simulink model "soc_dvbs2_top"  (R2025b)
settings: Solver=VariableStepAuto  StartTime=0.0  StopTime=0.3  RelTol=1e-3
PreLoadFcn:
  | RxFrameSize = 2048;
  | soc_dvbs2_init;
InitFcn:
  | RxFrameSize = 2048;
  | soc_dvbs2_init;
model workspace (MAT data in the model file):
  mmap = soc.memmap.MemoryMap
  mmap.isMapValid = 1
  mmap.controllerInfo = soc.memmap.MemController
  mmap.controllerInfo.memPSRange = {'2', 'G'}
  mmap.controllerInfo.memPLBaseAddr = '0x500000000'
  mmap.controllerInfo.memPLRange = {'4', 'G'}
  mmap.controllerInfo.memPLBaseAddrMMU = {9, '0'}
  mmap.controllerInfo.regBaseAddr = '0xA0000000'
  mmap.controllerInfo.regAddrRange = {'256', 'M'}
  mmap.map(1) = soc.memmap.MapParams
  mmap.map(1).type = 'PS Memory Region'
  mmap.map(1).name = 'AXI4-Stream to Software'
  mmap.map(1).baseAddr = '0x00000000'
  mmap.map(1).range = {'32', 'K'}
  mmap.map(1).path = 'soc_dvbs2_top/AXI4-Stream to Software'
  mmap.map(2) = soc.memmap.MapParams
  mmap.map(2).type = 'User Component'
  mmap.map(2).name = 'DVBS2'
  mmap.map(2).baseAddr = '0xA0000000'
  mmap.map(2).range = {'64', 'K'}
  mmap.map(2).path = 'soc_dvbs2_fpga/DVBS2'
  mmap.map(2).regs(1) = soc.memmap.IPCoreRegParams
  mmap.map(2).regs(1).register = 'HDL Coder registers'
  mmap.map(2).regs(1).offset = '0x0000 - 0x00FF'
  mmap.map(2).regs(1).vectorlength = 'N/A'
  mmap.map(2).regs(1).type = 'Reserved'
  mmap.map(2).regs(1).reserved = 1
  mmap.map(2).regs(2) = soc.memmap.IPCoreRegParams
  mmap.map(2).regs(2).blkname = 'DVBS2'
  mmap.map(2).regs(2).register = 'nframesSynced'
  mmap.map(2).regs(2).offset = '0x0100'
  mmap.map(2).regs(2).vectorlength = '1'
  mmap.map(2).regs(2).type = 'Processor read channel'
  mmap.map(2).regs(3) = soc.memmap.IPCoreRegParams
  mmap.map(2).regs(3).blkname = 'DVBS2'
  mmap.map(2).regs(3).register = 'decodedModcod'
  mmap.map(2).regs(3).offset = '0x0104'
  mmap.map(2).regs(3).vectorlength = '1'
  mmap.map(2).regs(3).type = 'Processor read channel'
  mmap.map(2).regs(4) = soc.memmap.IPCoreRegParams
  mmap.map(2).regs(4).blkname = 'DVBS2'
  mmap.map(2).regs(4).register = 'decodedFecFrame'
  mmap.map(2).regs(4).offset = '0x0108'
  mmap.map(2).regs(4).vectorlength = '1'
  mmap.map(2).regs(4).type = 'Processor read channel'
  mmap.map(2).regs(5) = soc.memmap.IPCoreRegParams
  mmap.map(2).regs(5).blkname = 'DVBS2'
  mmap.map(2).regs(5).register = 'FreqEst'
  mmap.map(2).regs(5).offset = '0x010C'
  mmap.map(2).regs(5).vectorlength = '1'
  mmap.map(2).regs(5).type = 'Processor read channel'
  mmap.map(2).regs(6) = soc.memmap.IPCoreRegParams
  mmap.map(2).regs(6).blkname = 'DVBS2'
  mmap.map(2).regs(6).register = 'TSorGS'
  mmap.map(2).regs(6).offset = '0x0110'
  mmap.map(2).regs(6).vectorlength = '1'
  mmap.map(2).regs(6).type = 'Processor read channel'
  mmap.map(2).regs(7) = soc.memmap.IPCoreRegParams
  mmap.map(2).regs(7).blkname = 'DVBS2'
  mmap.map(2).regs(7).register = 'UPL'
  mmap.map(2).regs(7).offset = '0x0114'
  mmap.map(2).regs(7).vectorlength = '1'
  mmap.map(2).regs(7).type = 'Processor read channel'
  mmap.map(2).regs(8) = soc.memmap.IPCoreRegParams
  mmap.map(2).regs(8).blkname = 'DVBS2'
  mmap.map(2).regs(8).register = 'DFL'
  mmap.map(2).regs(8).offset = '0x0118'
  mmap.map(2).regs(8).vectorlength = '1'
  mmap.map(2).regs(8).type = 'Processor read channel'
  mmap.map(2).regs(9) = soc.memmap.IPCoreRegParams
  mmap.map(2).regs(9).blkname = 'DVBS2'
  mmap.map(2).regs(9).register = 'SYNC'
  mmap.map(2).regs(9).offset = '0x011C'
  mmap.map(2).regs(9).vectorlength = '1'
  mmap.map(2).regs(9).type = 'Processor read channel'
  mmap.map(2).regs(10) = soc.memmap.IPCoreRegParams
  mmap.map(2).regs(10).blkname = 'DVBS2'
  mmap.map(2).regs(10).register = 'nbitsErrored'
  mmap.map(2).regs(10).offset = '0x0120'
  mmap.map(2).regs(10).vectorlength = '1'
  mmap.map(2).regs(10).type = 'Processor read channel'
  mmap.map(2).regs(11) = soc.memmap.IPCoreRegParams
  mmap.map(2).regs(11).blkname = 'DVBS2'
  mmap.map(2).regs(11).register = 'nbitsReceived'
  mmap.map(2).regs(11).offset = '0x0124'
  mmap.map(2).regs(11).vectorlength = '1'
  mmap.map(2).regs(11).type = 'Processor read channel'
  mmap.map(2).regs(12) = soc.memmap.IPCoreRegParams
  mmap.map(2).regs(12).blkname = 'DVBS2'
  mmap.map(2).regs(12).register = 'adc_dac_loopback'
  mmap.map(2).regs(12).offset = '0x0128'
  mmap.map(2).regs(12).vectorlength = '1'
  mmap.map(2).regs(12).type = 'Processor write channel'
  mmap.map(2).regs(13) = soc.memmap.IPCoreRegParams
  mmap.map(2).regs(13).blkname = 'DVBS2'
  mmap.map(2).regs(13).register = 'enbNoise'
  mmap.map(2).regs(13).offset = '0x012C'
  mmap.map(2).regs(13).vectorlength = '1'
  mmap.map(2).regs(13).type = 'Processor write channel'
  mmap.map(2).regs(14) = soc.memmap.IPCoreRegParams
  mmap.map(2).regs(14).blkname = 'DVBS2'
  mmap.map(2).regs(14).register = 'snrdB'
  mmap.map(2).regs(14).offset = '0x0130'
  mmap.map(2).regs(14).vectorlength = '1'
  mmap.map(2).regs(14).type = 'Processor write channel'
  mmap.map(2).regs(15) = soc.memmap.IPCoreRegParams
  mmap.map(2).regs(15).blkname = 'DVBS2'
  mmap.map(2).regs(15).register = 'CFO'
  mmap.map(2).regs(15).offset = '0x0134'
  mmap.map(2).regs(15).vectorlength = '1'
  mmap.map(2).regs(15).type = 'Processor write channel'
  mmap.map(2).regs(16) = soc.memmap.IPCoreRegParams
  mmap.map(2).regs(16).blkname = 'DVBS2'
  mmap.map(2).regs(16).register = 'CPO'
  mmap.map(2).regs(16).offset = '0x0138'
  mmap.map(2).regs(16).vectorlength = '1'
  mmap.map(2).regs(16).type = 'Processor write channel'
  mmap.map(2).regs(17) = soc.memmap.IPCoreRegParams
  mmap.map(2).regs(17).blkname = 'DVBS2'
  mmap.map(2).regs(17).register = 'modcodIdx'
  mmap.map(2).regs(17).offset = '0x013C'
  mmap.map(2).regs(17).vectorlength = '1'
  mmap.map(2).regs(17).type = 'Processor write channel'
  mmap.map(2).regs(18) = soc.memmap.IPCoreRegParams
  mmap.map(2).regs(18).blkname = 'DVBS2'
  mmap.map(2).regs(18).register = 'resetFCPO'
  mmap.map(2).regs(18).offset = '0x0140'
  mmap.map(2).regs(18).vectorlength = '1'
  mmap.map(2).regs(18).type = 'Processor write channel'
  mmap.map(2).regs(19) = soc.memmap.IPCoreRegParams
  mmap.map(2).regs(19).blkname = 'DVBS2'
  mmap.map(2).regs(19).register = 'resetDisplay'
  mmap.map(2).regs(19).offset = '0x0144'
  mmap.map(2).regs(19).vectorlength = '1'
  mmap.map(2).regs(19).type = 'Processor write channel'
  mmap.map(3) = soc.memmap.MapParams
  mmap.map(3).type = 'Implicit Component'
  mmap.map(3).name = 'AXI4-Stream to Software DMA S2MM'
  mmap.map(3).baseAddr = '0xA0010000'
  mmap.map(3).range = {'64', 'K'}
  mmap.map(4) = soc.memmap.MapParams
  mmap.map(4).type = 'Implicit Component'
  mmap.map(4).name = 'RFDataConverter/s_axi'
  mmap.map(4).baseAddr = '0xA3C00000'
  mmap.map(4).range = {'256', 'K'}
  mwTaskManagerKernelLatency = 0
  socicb{1}.Registry = containers.Map
  socicb{1}.Registry.serialization.keys = {45989.0006104}
  socicb{1}.Registry.serialization.values = {1}
  socicb{1}.Registry.serialization.uniformity = 0
  socicb{1}.Registry.serialization.keyType = 'double'
  socicb{1}.Registry.serialization.valueType = 'any'
  socicb{1}.Index = 2
  socicb{2}.Registry = containers.Map
  socicb{2}.Registry.serialization.keys = {}
  socicb{2}.Registry.serialization.values = {}
  socicb{2}.Registry.serialization.uniformity = 0
  socicb{2}.Registry.serialization.keyType = 'double'
  socicb{2}.Registry.serialization.valueType = 'any'
  socicb{2}.Index = 1
  socvcb = containers.Map
  socvcb.serialization.keys = {2.00012207031, 2.00024414062, 2.00036621094, 3.00012207031, 3.00036621094, 3.00061035156, 3.00073242188, 3.00109863281, 3.00158691406, 3.00219726562, 3.00329589844, 3.00366210938, 3.00939941406, 3.01062011719, 3.02478027344, 3.02746582031, 3.0302734375, 3.03332519531, 3.09558105469, 4.00012207031, 4.00024414062, 4.00036621094, 4.00061035156, 4.00073242188, 4.00109863281, 4.00122070312, 4.00183105469, 4.00891113281, 4.00915527344, 4.0244140625, 4.02673339844, 4.02807617188, 4.03259277344, 4.36804199219, 5.00061035156, 5.00073242188, 5.00122070312, 5.00134277344, 5.00891113281, 5.00915527344, 5.02429199219, 5.02648925781, 5.02734375, 5.03234863281, 154.00012207, 154.044311523, 154.045654297, 154.083618164, 154.113647461, 154.172729492, 155.003417969, 356.163696289, 514.000244141, 515.381347656, 515.829833984, 1542.00634766, 2562.56542969, 15856.0009766, 15857.0006104, 15858.0004883, 17279.0084229, 17280.0084229, 44819.0001221, 45026.0063477, 45722.0001221}
  socvcb.serialization.values : function handle (value not decoded)
  socvcb.serialization.uniformity = 0
  socvcb.serialization.keyType = 'double'
  socvcb.serialization.valueType = 'any'
values from neighbouring files (symbols this model uses):
  fs = Rsym *32    (= 128000000)    [soc_dvbs2_init.m]
undefined symbols (not defined in the file or in its folder): D1, Fs, I, m, n, P, Q
libraries: socmemlib x2, prociodatalib x2, hostiolib x2, proctasklib x1, xilinxrfsoclib x1
CloseFcn:
  | h = warning('off','MATLAB:rmpath:DirNotFound');
  | rmpath(fullfile(matlabroot,'toolbox','whdl','whdlexamples','whdlexamples'));
  | warning(h);
  | clear h;
settings Model: DataDictionary=dvbs2hdlReceiverData.sldd  SimulationMode=accelerator  Creator=The MathWorks, Inc.  LastModifiedBy=The MathWorks, Inc.
settings SolverCC: AlgebraicLoopSolver=TrustRegion  PositivePriorityOrder=on  AutoInsertRateTranBlk=on  MaxZcPerStep=1.0
settings DataIOCC: SaveFormat=StructureWithTime  ReturnWorkspaceOutputs=off
settings OptimizationCC: BlockReduction=off  ConditionallyExecuteInputs=off  DefaultParameterBehavior=Inlined  ReuseModelBlockBuffer=off  PassReuseOutputArgsAs=Individual arguments  MaxStackSize=64  EfficientTunableParamExpr=on
settings DebuggingCC: AlgebraicLoopMsg=error  SingleTaskRateTransMsg=error  IntegerOverflowMsg=none  ParameterPrecisionLossMsg=none  ParameterTunabilityLossMsg=error  UnconnectedInputMsg=warning  UnconnectedOutputMsg=warning  UnconnectedLineMsg=warning  SubsystemReferenceDiagnosticForUnitTest=warning  ArithmeticOperatorsInVariantConditions=warning
settings HardwareCC: ProdBitPerLong=64.0  ProdLargestAtomicInteger=LongLong  ProdLargestAtomicFloat=Double  ProdLongLongMode=on  ProdHWDeviceType=ARM Compatible->ARM Cortex-A (64-bit)  HardwareBoardFeatureSet=SoCBlockset
settings ModelReferenceCC: EnableRefExpFcnMdlSchedulingChecks=on  ModelReferenceNumInstancesAllowed=Single
settings SFSimCC: SimUseLocalCustomCode=off  CustomCodeUndefinedFunction=UseInterfaceOnly
settings RTWCC: SystemTargetFile=ert.tlc  HardwareBoard=Xilinx Zynq UltraScale+ RFSoC ZCU111 Evaluation Kit  TLCOptions="-aInlineSetEventsForThisBaseRateFcn=TLC_FALSE -aSuppressMultiTaskScheduler=TLC_FALSE  -aRateBasedStepFcn=0"  TemplateMakefile=ert_default_tmf  GenerateReport=on  RTWUseLocalCustomCode=off  Toolchain=Linaro AArch64 Linux v6.3.1  IncludeHyperlinkInReport=on  LaunchReport=on  GenerateTraceInfo=on  GenerateTraceReport=on  GenerateTraceReportSl=on  GenerateTraceReportSf=on  GenerateTraceReportEml=on  GPUComputeCapability=3.5  DLArmComputeVersion=19.05  Description=Embedded Coder
settings CodeAppCC: ForceParamTrailComments=on  IgnoreCustomStorageClasses=off  OperatorAnnotations=on  SimulinkDataObjDesc=on  SFDataObjDesc=on  InsertBlockDesc=on
settings ERTTargetCC: InlinedParameterPlacement=Hierarchical

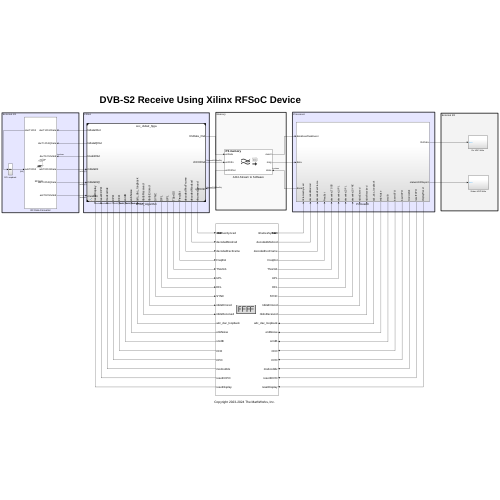
[thumbnail: Simulink's stored preview of the top-level diagram]
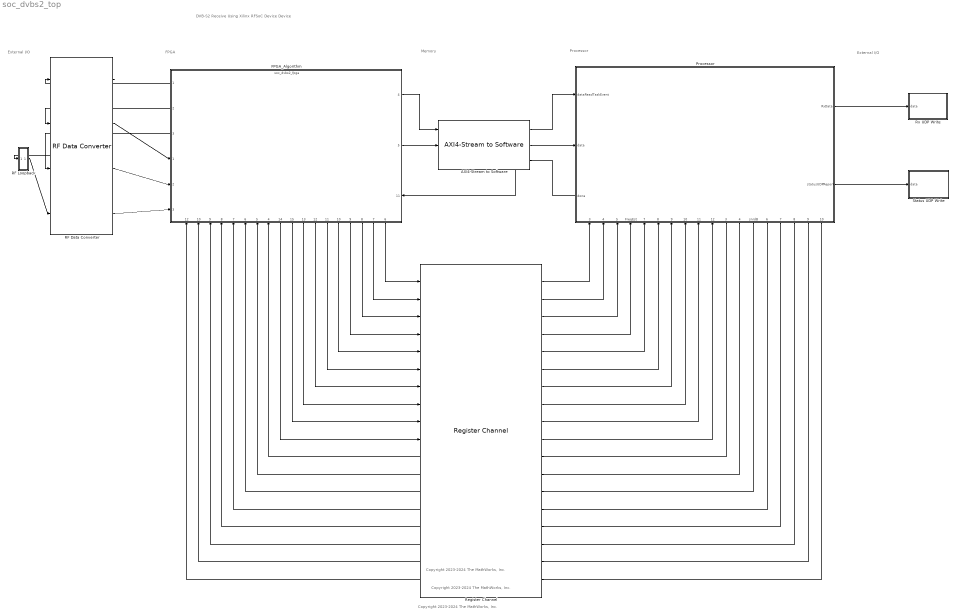
== system soc_dvbs2_top ==
  note: FPGA
  note: Memory
  note: Processor
  note: Copyright 2023-2024 The MathWorks, Inc.
  note: External I/O
  note: External I/O
  note: DVB-S2 Receive Using Xilinx RFSoC Device Device
  note: Copyright 2023-2024 The MathWorks, Inc.
  note: Copyright 2023-2024 The MathWorks, Inc.
  AXI4-Stream to Software : socmemlib/AXI4-Stream to Software  MemorySimulation=Burst accurate  MemorySelection=PS memory  MRNumBuffers=4  BurstLengthWriterChIf=256  FIFODepthWriter=8  FIFOAFullDepthWriter=6  ICClockFrequencyWriter=100  ICDataWidthWriter=64  ChDimensionsWriterChIf=1  ChTypeWriterChIf=uint32  ChFrameSampleTimeWriterChIf=1/fs  ChBitPackedWriterChIf=off  ChDimensionsReaderChIf=RxFrameSize  ChTypeReaderChIf=uint32  LastTargetBoard=Xilinx Zynq UltraScale+ RFSoC ZCU111 Evaluation Kit  MRRegionSize=32768  MRBufferSize=8192  DiagnosticLevel=No debug
  FPGA_Algorithm : ModelReference  ModelNameDialog=soc_dvbs2_fpga.slx  ModelReferenceVersion=9.0
      settings: PortSchema="{\"entries\":[{\"content\":{\"sides\":[{\"content\":{\"connectorIds\":[\"Out1\",\"Out2\",\"Out3\",\"In1\",\"In2\",\"In3\"]},\"type\":\"ConnectorPlacement.EquallySpacedRectSide\",\"uuid\":\"5a98e095-40d9-43f8-91e5-a805a03516fd\"},{\"content\":{\"connectorIds\":[\"Out4\",\"Out5\",\"In11\"],\"side\":\"RIGHT\"},\"type\":\"ConnectorPlacement.EquallySpacedRectSide\",\"uuid\":\"242f1ec7-c947-482c-82ab-d4fa225331bb\"},{\"content\":{\"side\":\"TOP\"},\"type\":\"ConnectorPlacement.EquallySpacedRectSide\",\"uuid\":\"d3f55be4-91f3-4b02-af75-0bf7e7e1b925\"},{\"content\":{\"connectorIds\":[\"In12\",\"In10\",\"In9\",\"In8\",\"In7\",\"In6\",\"In5\",\"In4\",\"Out14\",\"Out15\",\"Out13\",\"Out12\",\"Out11\",\"Out10\",\"Out9\",\"Out8\",\"Out7\",\"Out6\"],\"side\":\"BOTTOM\"},\"type\":\"ConnectorPlacement.EquallySpacedRectSide\",\"uuid\":\"11ee90da-1deb-4c1f-bd41-f9aa9c63736b\"}]},\"type\":\"ConnectorPlacement.EquallySpacedConnector\",\"uuid\":\"1ac0077b-1539-4750-8893-00c30e797fc3\"}],\"packageUris\":[\"http://schema.mathworks.com/mf0/Connector/R2020b\"],\"version\":\"1.0\"}"
  Processor : Subsystem
      settings: PortSchema="{\"entries\":[{\"content\":{\"sides\":[{\"content\":{\"connectorIds\":[\"In1\",\"In2\",\"Out11\"]},\"type\":\"ConnectorPlacement.EquallySpacedRectSide\",\"uuid\":\"19674b72-8bc7-450a-aa32-317c951772fa\"},{\"content\":{\"connectorIds\":[\"Out1\",\"Out2\"],\"side\":\"RIGHT\"},\"type\":\"ConnectorPlacement.EquallySpacedRectSide\",\"uuid\":\"8c37c977-a2a8-45d5-9785-0385e2fd1bd5\"},{\"content\":{\"side\":\"TOP\"},\"type\":\"ConnectorPlacement.EquallySpacedRectSide\",\"uuid\":\"969f5835-0601-41e1-8044-5c28f455717a\"},{\"content\":{\"connectorIds\":[\"In3\",\"In4\",\"In5\",\"In6\",\"In7\",\"In8\",\"In9\",\"In10\",\"In11\",\"In12\",\"Out3\",\"Out4\",\"Out5\",\"Out6\",\"Out7\",\"Out8\",\"Out9\",\"Out10\"],\"side\":\"BOTTOM\"},\"type\":\"ConnectorPlacement.EquallySpacedRectSide\",\"uuid\":\"78263d19-cd7e-4a64-923d-d1623dce68f9\"}]},\"type\":\"ConnectorPlacement.EquallySpacedConnector\",\"uuid\":\"9dca4fc9-649f-4a7f-a81c-0545d597adf9\"}],\"packageUris\":[\"http://schema.mathworks.com/mf0/Connector/R2020b\"],\"version\":\"1.0\"}"
  RF Data Converter : xilinxrfsoclib/RF Data Converter  RFDCSim=Pass-through  tabPromptsCB=0  RFInterface=Customize  digitalInterface=I/Q  dac11Enable=off  dac12Enable=off  dac13Enable=off  dac14Enable=off  dac21Enable=off  dac22Enable=off  dac23Enable=on  dac24Enable=off  dac31Enable=off  dac32Enable=off  dac33Enable=off  dac34Enable=off  dac41Enable=off  dac42Enable=off  dac43Enable=off  dac44Enable=off  matchDACParam=on  dacSampleRate=2048  dacDatapathMode=Full Nyquist (0 to Fs/2)  interpolationMode=4  dacSamplesPerCycle=4  dacMixerType=Fine  dacMixerMode=I/Q->Real  dacMixerFrequency=Fs/2  dacNCOFrequency=[0.860]  dacNCOPhase=[0]  invertSyncFilter=off  dacTile1SampleRate=1000  dac11DatapathMode=Full Nyquist (0 to Fs/2)  dac11InterpolationMode=2  dac11SamplesPerCycle=2  dac11MixerType=Coarse  dac11MixerMode=I/Q->Real  dac11MixerFrequency=Fs/2  dac11NCOFrequency=0  dac11NCOPhase=0  dac11InvertSyncFilter=off  dac12DatapathMode=Full Nyquist (0 to Fs/2)  dac12InterpolationMode=2  dac12SamplesPerCycle=2  dac12MixerType=Coarse  dac12MixerMode=I/Q->Real  dac12MixerFrequency=Fs/2  dac12NCOFrequency=0  dac12NCOPhase=0  dac12InvertSyncFilter=off  dac13DatapathMode=Full Nyquist (0 to Fs/2)  dac13InterpolationMode=2  dac13SamplesPerCycle=2  dac13MixerType=Coarse  dac13MixerMode=I/Q->Real  dac13MixerFrequency=Fs/2  dac13NCOFrequency=0  dac13NCOPhase=0  dac13InvertSyncFilter=off  dac14DatapathMode=Full Nyquist (0 to Fs/2)  dac14InterpolationMode=2  dac14SamplesPerCycle=2  dac14MixerType=Coarse  dac14MixerMode=I/Q->Real  dac14MixerFrequency=Fs/2  dac14NCOFrequency=0  dac14NCOPhase=0  dac14InvertSyncFilter=off  dacTile2SampleRate=1000  dac21DatapathMode=Full Nyquist (0 to Fs/2)  dac21InterpolationMode=2  dac21SamplesPerCycle=2  dac21MixerType=Coarse  dac21MixerMode=I/Q->Real  dac21MixerFrequency=Fs/2  dac21NCOFrequency=0  dac21NCOPhase=0  dac21InvertSyncFilter=off  dac22DatapathMode=Full Nyquist (0 to Fs/2)  dac22InterpolationMode=2  dac22SamplesPerCycle=2  dac22MixerType=Coarse  dac22MixerMode=I/Q->Real  dac22MixerFrequency=Fs/2  dac22NCOFrequency=0  dac22NCOPhase=0  dac22InvertSyncFilter=off  dac23DatapathMode=Full Nyquist (0 to Fs/2)  dac23InterpolationMode=2  dac23SamplesPerCycle=2  dac23MixerType=Coarse  dac23MixerMode=I/Q->Real  dac23MixerFrequency=Fs/2  dac23NCOFrequency=0  dac23NCOPhase=0  dac23InvertSyncFilter=off  dac24DatapathMode=Full Nyquist (0 to Fs/2)  dac24InterpolationMode=2  dac24SamplesPerCycle=2  dac24MixerType=Coarse  dac24MixerMode=I/Q->Real  dac24MixerFrequency=Fs/2  dac24NCOFrequency=0  dac24NCOPhase=0  dac24InvertSyncFilter=off  dacTile3SampleRate=1000  dac31DatapathMode=Full Nyquist (0 to Fs/2)  dac31InterpolationMode=2  dac31SamplesPerCycle=2  dac31MixerType=Coarse  dac31MixerMode=I/Q->Real  dac31MixerFrequency=Fs/2  dac31NCOFrequency=0  dac31NCOPhase=0  dac31InvertSyncFilter=off  dac32DatapathMode=Full Nyquist (0 to Fs/2)  dac32InterpolationMode=2  dac32SamplesPerCycle=2  dac32MixerType=Coarse  dac32MixerMode=I/Q->Real  dac32MixerFrequency=Fs/2  dac32NCOFrequency=0  dac32NCOPhase=0  dac32InvertSyncFilter=off  dac33DatapathMode=Full Nyquist (0 to Fs/2)  dac33InterpolationMode=2  dac33SamplesPerCycle=2  dac33MixerType=Coarse  dac33MixerMode=I/Q->Real  dac33MixerFrequency=Fs/2  dac33NCOFrequency=0  dac33NCOPhase=0  dac33InvertSyncFilter=off  dac34DatapathMode=Full Nyquist (0 to Fs/2)  dac34InterpolationMode=2  dac34SamplesPerCycle=2  dac34MixerType=Coarse  dac34MixerMode=I/Q->Real  dac34MixerFrequency=Fs/2  dac34NCOFrequency=0  dac34NCOPhase=0  dac34InvertSyncFilter=off  dacTile4SampleRate=1000  dac41DatapathMode=Full Nyquist (0 to Fs/2)  dac41InterpolationMode=2  dac41SamplesPerCycle=2  dac41MixerType=Coarse  dac41MixerMode=I/Q->Real  dac41MixerFrequency=Fs/2  dac41NCOFrequency=0  dac41NCOPhase=0  dac41InvertSyncFilter=off  dac42DatapathMode=Full Nyquist (0 to Fs/2)  dac42InterpolationMode=2  dac42SamplesPerCycle=2  dac42MixerType=Coarse  dac42MixerMode=I/Q->Real  dac42MixerFrequency=Fs/2  dac42NCOFrequency=0  dac42NCOPhase=0  dac42InvertSyncFilter=off  dac43DatapathMode=Full Nyquist (0 to Fs/2)  dac43InterpolationMode=2  dac43SamplesPerCycle=2  dac43MixerType=Coarse  dac43MixerMode=I/Q->Real  dac43MixerFrequency=Fs/2  dac43NCOFrequency=0  dac43NCOPhase=0  dac43InvertSyncFilter=off  dac44DatapathMode=Full Nyquist (0 to Fs/2)  dac44InterpolationMode=2  dac44SamplesPerCycle=2  dac44MixerType=Coarse  dac44MixerMode=I/Q->Real  dac44MixerFrequency=Fs/2  dac44NCOFrequency=0  dac44NCOPhase=0  dac44InvertSyncFilter=off  adc11Enable=on  adc12Enable=off  adc13Enable=off  adc14Enable=off  adc21Enable=off  adc22Enable=off  adc23Enable=off  adc24Enable=off  adc31Enable=off  adc32Enable=off  adc33Enable=off  adc34Enable=off  adc41Enable=off  adc42Enable=off  adc43Enable=off  adc44Enable=off  adcOutUnpackedData=on  matchADCParam=on  adcSampleRate=2048  decimationMode=4  adcSamplesPerCycle=4  adcMixerType=Fine  adcMixerMode=Real->I/Q  adcMixerFrequency=Fs/2  adcNCOFrequency=[-0.860]  adcNCOPhase=[0]  adcTile1SampleRate=1000  adc11DecimationMode=2  adc11SamplesPerCycle=2  adc11MixerType=Coarse  adc11MixerMode=Real->I/Q  adc11MixerFrequency=Fs/2  adc11NCOFrequency=0  adc11NCOPhase=0  adc12DecimationMode=2  adc12SamplesPerCycle=2  adc12MixerType=Coarse  adc12MixerMode=Real->I/Q  adc12MixerFrequency=Fs/2  adc12NCOFrequency=0  adc12NCOPhase=0  adc13DecimationMode=2  adc13SamplesPerCycle=2  adc13MixerType=Coarse  adc13MixerMode=Real->I/Q  adc13MixerFrequency=Fs/2  adc13NCOFrequency=0  adc13NCOPhase=0  adc14DecimationMode=2  adc14SamplesPerCycle=2  adc14MixerType=Coarse  adc14MixerMode=Real->I/Q  adc14MixerFrequency=Fs/2  adc14NCOFrequency=0  adc14NCOPhase=0  adcTile2SampleRate=1000  adc21DecimationMode=2  adc21SamplesPerCycle=2  adc21MixerType=Coarse  adc21MixerMode=Real->I/Q  adc21MixerFrequency=Fs/2  adc21NCOFrequency=0  adc21NCOPhase=0  adc22DecimationMode=2  adc22SamplesPerCycle=2  adc22MixerType=Coarse  adc22MixerMode=Real->I/Q  adc22MixerFrequency=Fs/2  adc22NCOFrequency=0  adc22NCOPhase=0  adc23DecimationMode=2  adc23SamplesPerCycle=2  adc23MixerType=Coarse  adc23MixerMode=Real->I/Q  adc23MixerFrequency=Fs/2  adc23NCOFrequency=0  adc23NCOPhase=0  adc24DecimationMode=2  adc24SamplesPerCycle=2  adc24MixerType=Coarse  adc24MixerMode=Real->I/Q  adc24MixerFrequency=Fs/2  adc24NCOFrequency=0  adc24NCOPhase=0  adcTile3SampleRate=1000  adc31DecimationMode=2  adc31SamplesPerCycle=2  adc31MixerType=Coarse  adc31MixerMode=Real->I/Q  adc31MixerFrequency=Fs/2  adc31NCOFrequency=0  adc31NCOPhase=0  adc32DecimationMode=2  adc32SamplesPerCycle=2  adc32MixerType=Coarse  adc32MixerMode=Real->I/Q  adc32MixerFrequency=Fs/2  adc32NCOFrequency=0  adc32NCOPhase=0  adc33DecimationMode=2  adc33SamplesPerCycle=2  adc33MixerType=Coarse  adc33MixerMode=Real->I/Q  adc33MixerFrequency=Fs/2  adc33NCOFrequency=0  adc33NCOPhase=0  adc34DecimationMode=2  adc34SamplesPerCycle=2  adc34MixerType=Coarse  adc34MixerMode=Real->I/Q  adc34MixerFrequency=Fs/2  adc34NCOFrequency=0  adc34NCOPhase=0  adcTile4SampleRate=1000  adc41DecimationMode=2  adc41SamplesPerCycle=2  adc41MixerType=Coarse  adc41MixerMode=Real->I/Q  adc41MixerFrequency=Fs/2  adc41NCOFrequency=0  adc41NCOPhase=0  adc42DecimationMode=2  adc42SamplesPerCycle=2  adc42MixerType=Coarse  adc42MixerMode=Real->I/Q  adc42MixerFrequency=Fs/2  adc42NCOFrequency=0  adc42NCOPhase=0  adc43DecimationMode=2  adc43SamplesPerCycle=2  adc43MixerType=Coarse  adc43MixerMode=Real->I/Q  adc43MixerFrequency=Fs/2  adc43NCOFrequency=0  adc43NCOPhase=0  adc44DecimationMode=2  adc44SamplesPerCycle=2  adc44MixerType=Coarse  adc44MixerMode=Real->I/Q  adc44MixerFrequency=Fs/2  adc44NCOFrequency=0  adc44NCOPhase=0  multiTileSync=off  externalPLL=off  dacRealTimeNCOPortsEnable=off  adcRealTimeNCOPortsEnable=off  adcRealTimePortsEnable=off  adcThresholdMode=Sticky over  adcThreshold1=0  adcDelayCounter=0  adcThreshold2Mode=Sticky over  adcThreshold2=0  adcThreshold2DelayCounter=0  adc11ThresholdMode=Sticky over  adc11Threshold1=0  adc11DelayCounter=0  adc11Threshold2Mode=Sticky over  adc11Threshold2=0  adc11Threshold2DelayCounter=0  adc12ThresholdMode=Sticky over  adc12Threshold1=0  adc12DelayCounter=0  adc12Threshold2Mode=Sticky over  adc12Threshold2=0  adc12Threshold2DelayCounter=0  adc13ThresholdMode=Sticky over  adc13Threshold1=0  adc13DelayCounter=0  adc13Threshold2Mode=Sticky over  adc13Threshold2=0  adc13Threshold2DelayCounter=0  adc14ThresholdMode=Sticky over  adc14Threshold1=0  adc14DelayCounter=0  adc14Threshold2Mode=Sticky over  adc14Threshold2=0  adc14Threshold2DelayCounter=0  adc21ThresholdMode=Sticky over  adc21Threshold1=0  adc21DelayCounter=0  adc21Threshold2Mode=Sticky over  adc21Threshold2=0  adc21Threshold2DelayCounter=0  adc22ThresholdMode=Sticky over  adc22Threshold1=0  adc22DelayCounter=0  adc22Threshold2Mode=Sticky over  adc22Threshold2=0  adc22Threshold2DelayCounter=0  adc23ThresholdMode=Sticky over  adc23Threshold1=0  adc23DelayCounter=0  adc23Threshold2Mode=Sticky over  adc23Threshold2=0  adc23Threshold2DelayCounter=0  adc24ThresholdMode=Sticky over  adc24Threshold1=0  adc24DelayCounter=0  adc24Threshold2Mode=Sticky over  adc24Threshold2=0  adc24Threshold2DelayCounter=0  adc31ThresholdMode=Sticky over  adc31Threshold1=0  adc31DelayCounter=0  adc31Threshold2Mode=Sticky over  adc31Threshold2=0  adc31Threshold2DelayCounter=0  adc32ThresholdMode=Sticky over  adc32Threshold1=0  adc32DelayCounter=0  adc32Threshold2Mode=Sticky over  adc32Threshold2=0  adc32Threshold2DelayCounter=0  adc33ThresholdMode=Sticky over  adc33Threshold1=0  adc33DelayCounter=0  adc33Threshold2Mode=Sticky over  adc33Threshold2=0  adc33Threshold2DelayCounter=0  adc34ThresholdMode=Sticky over  adc34Threshold1=0  adc34DelayCounter=0  adc34Threshold2Mode=Sticky over  adc34Threshold2=0  adc34Threshold2DelayCounter=0  adc41ThresholdMode=Sticky over  adc41Threshold1=0  adc41DelayCounter=0  adc41Threshold2Mode=Sticky over  adc41Threshold2=0  adc41Threshold2DelayCounter=0  adc42ThresholdMode=Sticky over  adc42Threshold1=0  adc42DelayCounter=0  adc42Threshold2Mode=Sticky over  adc42Threshold2=0  adc42Threshold2DelayCounter=0  adc43ThresholdMode=Sticky over  adc43Threshold1=0  adc43DelayCounter=0  adc43Threshold2Mode=Sticky over  adc43Threshold2=0  adc43Threshold2DelayCounter=0  adc44ThresholdMode=Sticky over  adc44Threshold1=0  adc44DelayCounter=0  adc44Threshold2Mode=Sticky over  adc44Threshold2=0  adc44Threshold2DelayCounter=0
  RF Loopback : Subsystem
  Register Channel : socmemlib/Register Channel  RegisterTable={ 'nframesSynced', 'Read', 'uint32', '1'; 'decodedModcod', 'Read', 'fixdt(0,5,0)', '1'; 'decodedFecFrame', 'Read', 'fixdt(0,1,0)', '1'; 'FreqEst', 'Read', 'fixdt(1,21,21)', '1'; 'TSorGS', 'Read', 'fixdt(0,2,0)', '1'; 'UPL', 'Read', 'uint16', '1'; 'DFL', 'Read', 'uint16', '1'; 'SYNC', 'Read', 'uint8', '1'; 'nbitsErrored', 'Read', 'uint32', '1'; 'nbitsReceived', 'Read', 'uint32', '1'; 'adc_dac_loopback', 'Write', 'boolean', '1'; 'enbNoise', 'Write', 'boolean', '1'; 'snrdB', 'Write', 'fixdt(1,16,9)', '1'; 'CFO', 'Write', 'fixdt(1,21,21)', '1'; 'CPO', 'Write', 'fixdt(1,21,21)', '1'; 'modcodIdx', 'Write', 'fixdt(0,5,0)', '1'; 'resetFCPO', 'Write', 'boolean', '1'; 'resetDisplay', 'Write', 'boolean', '1' }  SampleTime=1/fs  RegTableNames={'nframesSynced' 'decodedModcod' 'decodedFecFrame' 'FreqEst' 'TSorGS' 'UPL' 'DFL' 'SYNC' 'nbitsErrored' 'nbitsReceived' 'adc_dac_loopback' 'enbNoise' 'snrdB' 'CFO' 'CPO' 'modcodIdx' 'resetFCPO' 'resetDisplay' }  RegTableRW={'Read' 'Read' 'Read' 'Read' 'Read' 'Read' 'Read' 'Read' 'Read' 'Read' 'Write' 'Write' 'Write' 'Write' 'Write' 'Write' 'Write' 'Write' }  RegTableDataTypes={'uint32' 'fixdt(0,5,0)' 'fixdt(0,1,0)' 'fixdt(1,21,21)' 'fixdt(0,2,0)' 'uint16' 'uint16' 'uint8' 'uint32' 'uint32' 'boolean' 'boolean' 'fixdt(1,16,9)' 'fixdt(1,21,21)' 'fixdt(1,21,21)' 'fixdt(0,5,0)' 'boolean' 'boolean' }  RegTableVectorSizes={'1' '1' '1' '1' '1' '1' '1' '1' '1' '1' '1' '1' '1' '1' '1' '1' '1' '1' }  NumRegisters=18  RegTableInitialValues={'0','0','0','0','0','0','0','0','0','0','0','0','0','0','0','0','0','0'}  RegTableDirty=0
  Rx UDP Write : Subsystem
  Status UDP Write : Subsystem
  wires:
  RF Data Converter/2 -> FPGA_Algorithm/1
  RF Data Converter/1 -> RF Loopback/1(dac)
  FPGA_Algorithm/1 -> RF Data Converter/1
  FPGA_Algorithm/3 -> RF Data Converter/3
  FPGA_Algorithm/2 -> RF Data Converter/2
  RF Data Converter/3 -> FPGA_Algorithm/2
  Processor/2(statusUDPReport) -> Status UDP Write/1(data)
  RF Loopback/1(adc) -> RF Data Converter/4
  Processor/1(RxData) -> Rx UDP Write/1(data)
  RF Data Converter/4 -> FPGA_Algorithm/3
  Processor/11(done) -> AXI4-Stream to Software/3
  AXI4-Stream to Software/2 -> Processor/2(data)
  AXI4-Stream to Software/1 -> Processor/1(dataReadTaskEvent)
  FPGA_Algorithm/4 -> AXI4-Stream to Software/1
  FPGA_Algorithm/5 -> AXI4-Stream to Software/2
  AXI4-Stream to Software/3 -> FPGA_Algorithm/11
  FPGA_Algorithm/6 -> Register Channel/1
  FPGA_Algorithm/7 -> Register Channel/2
  FPGA_Algorithm/8 -> Register Channel/3
  FPGA_Algorithm/9 -> Register Channel/4
  FPGA_Algorithm/10 -> Register Channel/5
  FPGA_Algorithm/11 -> Register Channel/6
  FPGA_Algorithm/12 -> Register Channel/7
  FPGA_Algorithm/13 -> Register Channel/8
  Register Channel/1 -> Processor/3(nFramesSynced)
  Register Channel/2 -> Processor/4(decodedModcod)
  Register Channel/3 -> Processor/5(decodedFecFrame)
  FPGA_Algorithm/15 -> Register Channel/9
  FPGA_Algorithm/14 -> Register Channel/10
  Register Channel/11 -> FPGA_Algorithm/4
  Register Channel/12 -> FPGA_Algorithm/5
  Register Channel/13 -> FPGA_Algorithm/6
  Register Channel/14 -> FPGA_Algorithm/7
  Register Channel/15 -> FPGA_Algorithm/8
  Register Channel/16 -> FPGA_Algorithm/9
  Register Channel/17 -> FPGA_Algorithm/10
  Register Channel/18 -> FPGA_Algorithm/12
  Register Channel/4 -> Processor/6(FreqEst)
  Register Channel/5 -> Processor/7(decoded_TSGS)
  Register Channel/6 -> Processor/8(decoded_UPL)
  Register Channel/7 -> Processor/9(decoded_DFL)
  Register Channel/8 -> Processor/10(decoded_SYNC)
  Register Channel/9 -> Processor/11(nbitsErrored)
  Register Channel/10 -> Processor/12(nbitsReceived)
  Processor/3(adc_dac_loopback) -> Register Channel/11
  Processor/4(enbNoise) -> Register Channel/12
  Processor/5(snrdB) -> Register Channel/13
  Processor/6(insertCFO) -> Register Channel/14
  Processor/7(insertCPO) -> Register Channel/15
  Processor/8(modcodIdx) -> Register Channel/16
  Processor/9(resetFCPO) -> Register Channel/17
  Processor/10(displayReset) -> Register Channel/18

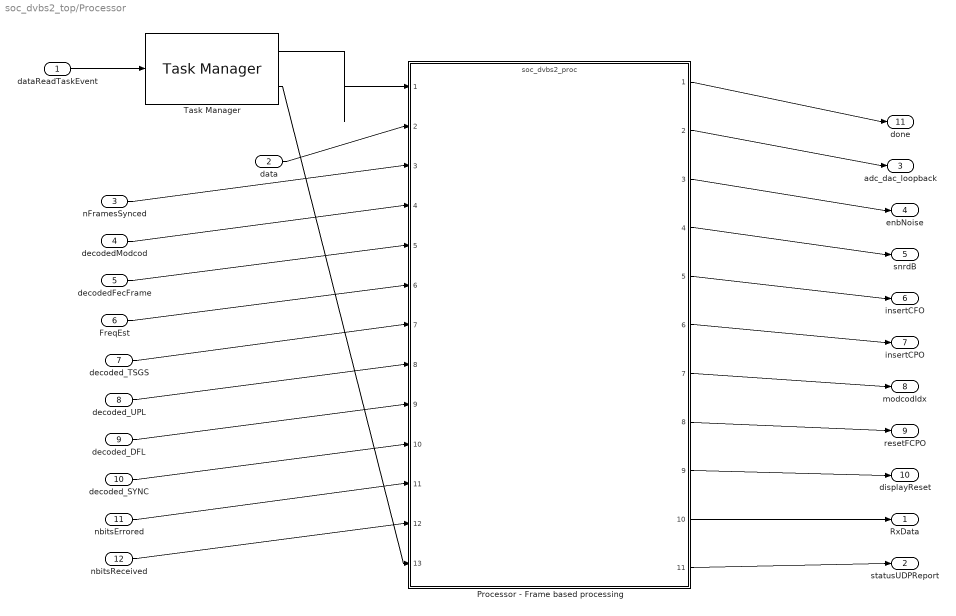
== system soc_dvbs2_top/Processor ==
  dataReadTaskEvent : Inport
  data : Inport  Port=2
  nFramesSynced : Inport  Port=3
  decodedModcod : Inport  Port=4
  decodedFecFrame : Inport  Port=5
  FreqEst : Inport  Port=6
  decoded_TSGS : Inport  Port=7
  decoded_UPL : Inport  Port=8
  decoded_DFL : Inport  Port=9
  decoded_SYNC : Inport  Port=10
  nbitsErrored : Inport  Port=11
  nbitsReceived : Inport  Port=12
  Processor - Frame based processing : ModelReference  InputPortMessageModes=n,m,m,m,m,m,m,m,m,m,m,m,n  OutputPortMessageModes=m,m,m,m,m,m,m,m,m,m,m  ModelNameDialog=soc_dvbs2_proc.slx  SimulationMode=Normal  ScheduleRates=on  CachedPortDiscreteRates=[0.001]  ModelEventPortInfo=P:D1[0.001][0][0]  ModelReferenceVersion=11.0
  Task Manager : proctasklib/Task Manager  AllTaskData="[{\"taskName\":\"dataReadTask\",\"taskType\":\"Event-driven\",\"taskEvent\":\"dataReadTaskEvent\",\"taskPeriod\":\"0.1\",\"taskPriority\":\"50\",\"coreSelection\":\"Specified core\",\"coreNum\":\"0\",\"dropOverranTasks\":false,\"playbackRecorded\":false,\"diagnosticsFile\":\"\",\"taskDurationSource\":\"Dialog\",\"taskDuration\":1E-6,\"taskDurationDeviation\":0,\"logExecutionData\":true,\"logDroppedTasks\":false,\"version\":\"2.6\",\"taskDurationData\":{\"percent\":[\"100\"],\"mean\":[\"1e-06\"],\"dev\":[\"0\"],\"min\":[\"1e-06\"],\"max\":[\"1e-06\"]},\"taskEventSource\":\"AXI4-Stream to Software\",\"taskEventSourceAssignmentType\":\"AutoAssigned\",\"taskEventSourceType\":\"Stream\",\"taskEventGroup\":\"Unspecified\",\"taskEventInterrupt\":\"Unspecified\",\"taskEventOrder\":1,\"taskDisablePremption\":false,\"taskClearInterruptFlagsAtEndOfEvent\":false},{\"taskName\":\"Periodic\",\"taskType\":\"Timer-driven\",\"taskEvent\":\"PeriodicEvent\",\"taskPeriod\":\"1e-3\",\"taskPriority\":\"51\",\"coreSelection\":\"Specified core\",\"coreNum\":\"0\",\"dropOverranTasks\":false,\"playbackRecorded\":false,\"diagnosticsFile\":\"\",\"taskDurationSource\":\"Dialog\",\"taskDuration\":1E-6,\"taskDurationDeviation\":0,\"logExecutionData\":true,\"logDroppedTasks\":false,\"version\":\"2.6\",\"taskDurationData\":{\"percent\":[\"100\"],\"mean\":[\"1e-06\"],\"dev\":[\"0\"],\"min\":[\"1e-06\"],\"max\":[\"1e-06\"]},\"taskEventSource\":\"Internal\",\"taskEventSourceAssignmentType\":\"AutoAssigned\",\"taskEventSourceType\":\"Unspecified\",\"taskEventGroup\":\"Unspecified\",\"taskEventInterrupt\":\"Unspecified\",\"taskEventOrder\":1,\"taskDisablePremption\":false,\"taskClearInterruptFlagsAtEndOfEvent\":false}]"  EnableTaskSimulation=on  StreamToSDI=on  WriteToFile=off  OverwriteFile=off  SupportEventPorts=on  UseScheduleEditor=off  CustomizationInfo=''
  RxData : Outport
  statusUDPReport : Outport  Port=2
  adc_dac_loopback : Outport  Port=3
  enbNoise : Outport  Port=4
  snrdB : Outport  Port=5
  insertCFO : Outport  Port=6
  insertCPO : Outport  Port=7
  modcodIdx : Outport  Port=8
  resetFCPO : Outport  Port=9
  displayReset : Outport  Port=10
  done : Outport  Port=11
  wires:
  dataReadTaskEvent/1 -> Task Manager/1
  data/1 -> Processor - Frame based processing/2
  Processor - Frame based processing/1 -> done/1
  Processor - Frame based processing/2 -> adc_dac_loopback/1
  Task Manager/1 -> Processor - Frame based processing/1
  Processor - Frame based processing/11 -> statusUDPReport/1
  Task Manager/2 -> Processor - Frame based processing/13
  nFramesSynced/1 -> Processor - Frame based processing/3
  decodedModcod/1 -> Processor - Frame based processing/4
  decodedFecFrame/1 -> Processor - Frame based processing/5
  Processor - Frame based processing/3 -> enbNoise/1
  Processor - Frame based processing/4 -> snrdB/1
  Processor - Frame based processing/5 -> insertCFO/1
  Processor - Frame based processing/6 -> insertCPO/1
  Processor - Frame based processing/7 -> modcodIdx/1
  Processor - Frame based processing/8 -> resetFCPO/1
  Processor - Frame based processing/9 -> displayReset/1
  Processor - Frame based processing/10 -> RxData/1
  nbitsErrored/1 -> Processor - Frame based processing/11
  nbitsReceived/1 -> Processor - Frame based processing/12
  decoded_SYNC/1 -> Processor - Frame based processing/10
  decoded_DFL/1 -> Processor - Frame based processing/9
  decoded_UPL/1 -> Processor - Frame based processing/8
  decoded_TSGS/1 -> Processor - Frame based processing/7
  FreqEst/1 -> Processor - Frame based processing/6

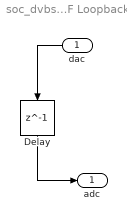
== system soc_dvbs2_top/RF Loopback ==
  dac : Inport
  Delay : Delay  DelayLength=1
  adc : Outport
  wires:
  dac/1 -> Delay/1
  Delay/1 -> adc/1

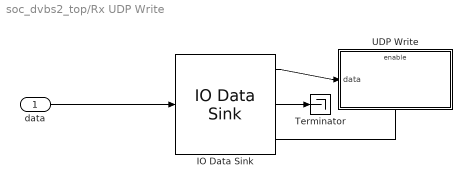
== system soc_dvbs2_top/Rx UDP Write ==
  data : Inport
  IO Data Sink : prociodatalib/IO Data Sink  OutputSink=To output port  DataTypeStr=uint32  Dimensions=RxFrameSize  DeviceType=UDP  EventDataPort=Data  QueueLength=65535  SampleTime=0.001  EnableDonePort=off
  Terminator : Terminator
  "UDP Write " : Subsystem
  wires:
  IO Data Sink/1 -> "UDP Write "/1(data)
  IO Data Sink/2 -> Terminator/1
  IO Data Sink/3 -> "UDP Write "/Enable
  data/1 -> IO Data Sink/1

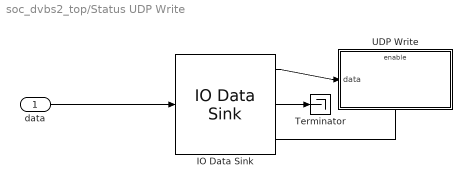
== system soc_dvbs2_top/Status UDP Write ==
  data : Inport
  IO Data Sink : prociodatalib/IO Data Sink  OutputSink=To output port  DataTypeStr=uint32  Dimensions=10  DeviceType=UDP  EventDataPort=Data  QueueLength=65535  SampleTime=0.001  EnableDonePort=off
  Terminator : Terminator
  "UDP Write " : Subsystem
  wires:
  IO Data Sink/1 -> "UDP Write "/1(data)
  IO Data Sink/2 -> Terminator/1
  IO Data Sink/3 -> "UDP Write "/Enable
  data/1 -> IO Data Sink/1

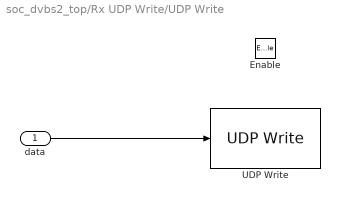
== system soc_dvbs2_top/Rx UDP Write/UDP Write  ==
  data : Inport
  Enable : EnablePort
  UDP Write : hostiolib/UDP Write  remoteURL='255.255.255.255'  remotePort=25000  localURL='255.255.255.255'  localPortSource=Automatically determine  localPort=-1  sampletime=-1  separateLengthPort=0  blockPlatform=HOST  hoistedMaskSrc=UDP Write/UDP Write Sim/UDP Write
  wires:
  data/1 -> UDP Write/1

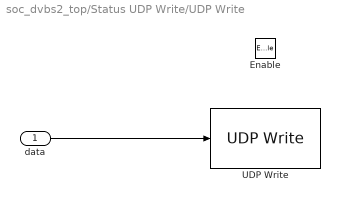
== system soc_dvbs2_top/Status UDP Write/UDP Write  ==
  data : Inport
  Enable : EnablePort
  UDP Write : hostiolib/UDP Write  remoteURL='255.255.255.255'  remotePort=25001  localURL='255.255.255.255'  localPortSource=Automatically determine  localPort=-1  sampletime=-1  separateLengthPort=0  blockPlatform=HOST  hoistedMaskSrc=UDP Write/UDP Write Sim/UDP Write
  wires:
  data/1 -> UDP Write/1
